simulink model "ng_pv_dynamic_dbus_p_4_ss_pmu"  (Simulink 8.8)
settings: Solver=ode4  StartTime=0.0  StopTime=inf  FixedStep=0.000125  RelTol=1e-3  EnableMultiTasking=on
PreLoadFcn:
  | Ts=125e-6;Core_Num = 0; np=1; nq=1; Vmin=.9;
PostLoadFcn:
  | Ts=125e-6;Core_Num = 0; np=1; nq=1; Vmin=.9;
InitFcn:
  | Ts=125e-6;Core_Num = 0; np=1; nq=1; Vmin=.9;
libraries: powerlib_meascontrol x180, rtio_generic_c37_118 x22, simulink x22, opal_lib x4, artemis x1, rtlab x1, powerlib x1
(part 4 of 4)

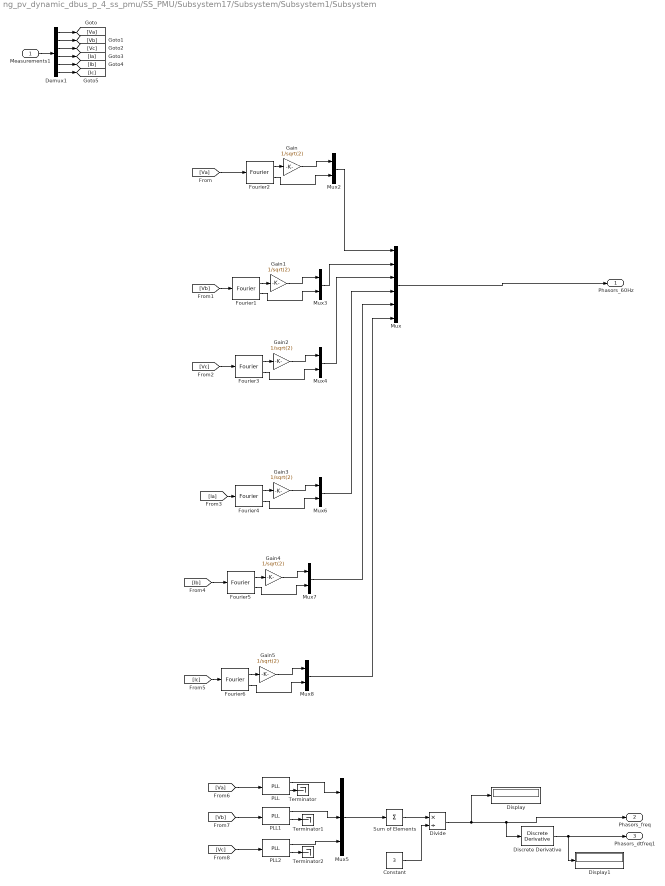
== system ng_pv_dynamic_dbus_p_4_ss_pmu/SS_PMU/Subsystem17/Subsystem/Subsystem1/Subsystem ==
  Measurements1 : Inport
  Constant : Constant  Value=3
  Demux1 : Demux  Outputs=6
  Discrete Derivative : simulink/Discrete/Discrete Derivative  gainval=1.0  ICPrevScaledInput=0.0  InputProcessing=Inherited  OutMin=[]  OutMax=[]  OutDataType=fixdt(1, 16)  OutScaling=2^-10  DoSatur=off
  Display : Display
  Display1 : Display
  Divide : Product  Inputs=*/
  Fourier{1..6} (6 alike) : powerlib_meascontrol/Measurements/Fourier  Freq=60  n=1  InInit=[0, 0]  Ts=Ts
  Gain{,1..5} (6 alike) : Gain  Gain=1/sqrt(2)
  Mux : Mux  Inputs=6
  Mux{2..4,6..8} (6 alike) : Mux  Inputs=2
  Mux5 : Mux  Inputs=3
  PLL : powerlib_meascontrol/PLL/PLL  Fmin=60  Par_Init=[0, 60]  ParK=[180, 3200, 1]  TcD=1.6e-4  MaxRateChangeFreq=12  FilterCutOffFreq=25  Ts=Ts  AGC=on
  PLL1 : powerlib_meascontrol/PLL/PLL  Fmin=60  Par_Init=[0, 60]  ParK=[180, 3200, 1]  TcD=1.6e-4  MaxRateChangeFreq=12  FilterCutOffFreq=25  Ts=Ts  AGC=on
  PLL2 : powerlib_meascontrol/PLL/PLL  Fmin=60  Par_Init=[0, 60]  ParK=[180, 3200, 1]  TcD=1.6e-4  MaxRateChangeFreq=12  FilterCutOffFreq=25  Ts=Ts  AGC=on
  Sum of Elements : Sum  Inputs=+
  Terminator : Terminator
  Terminator1 : Terminator
  Terminator2 : Terminator
  Phasors_60Hz : Outport
  Phasors_freq : Outport  Port=2
  Phasors_dtfreq1 : Outport  Port=3
  wires:
  Mux5/1 -> Sum of Elements/1
  PLL2/1 -> Mux5/3
  PLL1/1 -> Mux5/2
  PLL/1 -> Mux5/1
  PLL2/2 -> Terminator2/1
  PLL1/2 -> Terminator1/1
  PLL/2 -> Terminator/1
  [Vc] -> PLL2/1
  [Vb] -> PLL1/1
  [Va] -> PLL/1
  Discrete Derivative/1 -> Display1/1, Phasors_dtfreq1/1
  Mux3/1 -> Mux/2
  Mux2/1 -> Mux/1
  Demux1/2 -> [Vb]
  Measurements1/1 -> Demux1/1
  [Va] -> Fourier2/1
  Demux1/3 -> [Vc]
  Demux1/1 -> [Va]
  Mux7/1 -> Mux/5
  Mux4/1 -> Mux/3
  Mux/1 -> Phasors_60Hz/1
  Demux1/4 -> [Ia]
  Demux1/6 -> [Ic]
  Demux1/5 -> [Ib]
  Mux8/1 -> Mux/6
  Mux6/1 -> Mux/4
  Sum of Elements/1 -> Divide/1
  Divide/1 -> Display/1, Discrete Derivative/1, Phasors_freq/1
  Constant/1 -> Divide/2
  Fourier2/2 -> Mux2/2
  [Vc] -> Fourier3/1
  [Ia] -> Fourier4/1
  Fourier2/1 -> Gain/1
  Gain/1 -> Mux2/1
  [Vb] -> Fourier1/1
  Fourier1/2 -> Mux3/2
  Fourier1/1 -> Gain1/1
  Gain1/1 -> Mux3/1
  Fourier3/2 -> Mux4/2
  Fourier3/1 -> Gain2/1
  Gain2/1 -> Mux4/1
  Fourier4/2 -> Mux6/2
  Fourier4/1 -> Gain3/1
  Gain3/1 -> Mux6/1
  Fourier5/2 -> Mux7/2
  Fourier5/1 -> Gain4/1
  Gain4/1 -> Mux7/1
  Fourier6/2 -> Mux8/2
  Fourier6/1 -> Gain5/1
  Gain5/1 -> Mux8/1
  [Ic] -> Fourier6/1
  [Ib] -> Fourier5/1

== system ng_pv_dynamic_dbus_p_4_ss_pmu/SS_PMU/Subsystem18/Subsystem/Subsystem1/Degree to radian1 ==
  Degree : Inport
  Constant : Constant  Value=pi
  Constant1 : Constant  Value=180
  Divide : Product  Inputs=*/
  Product : Product  RndMeth=Zero
  Radian : Outport
  wires:
  Divide/1 -> Radian/1
  Degree/1 -> Product/1
  Constant1/1 -> Divide/2
  Product/1 -> Divide/1
  Constant/1 -> Product/2

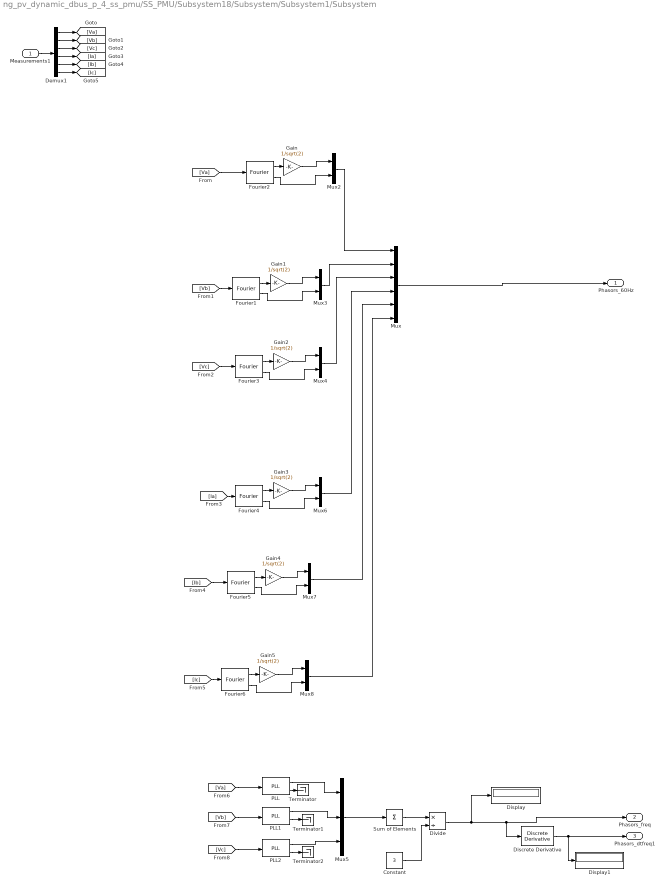
== system ng_pv_dynamic_dbus_p_4_ss_pmu/SS_PMU/Subsystem18/Subsystem/Subsystem1/Subsystem ==
  Measurements1 : Inport
  Constant : Constant  Value=3
  Demux1 : Demux  Outputs=6
  Discrete Derivative : simulink/Discrete/Discrete Derivative  gainval=1.0  ICPrevScaledInput=0.0  InputProcessing=Inherited  OutMin=[]  OutMax=[]  OutDataType=fixdt(1, 16)  OutScaling=2^-10  DoSatur=off
  Display : Display
  Display1 : Display
  Divide : Product  Inputs=*/
  Fourier{1..6} (6 alike) : powerlib_meascontrol/Measurements/Fourier  Freq=60  n=1  InInit=[0, 0]  Ts=Ts
  Gain{,1..5} (6 alike) : Gain  Gain=1/sqrt(2)
  Mux : Mux  Inputs=6
  Mux{2..4,6..8} (6 alike) : Mux  Inputs=2
  Mux5 : Mux  Inputs=3
  PLL : powerlib_meascontrol/PLL/PLL  Fmin=60  Par_Init=[0, 60]  ParK=[180, 3200, 1]  TcD=1.6e-4  MaxRateChangeFreq=12  FilterCutOffFreq=25  Ts=Ts  AGC=on
  PLL1 : powerlib_meascontrol/PLL/PLL  Fmin=60  Par_Init=[0, 60]  ParK=[180, 3200, 1]  TcD=1.6e-4  MaxRateChangeFreq=12  FilterCutOffFreq=25  Ts=Ts  AGC=on
  PLL2 : powerlib_meascontrol/PLL/PLL  Fmin=60  Par_Init=[0, 60]  ParK=[180, 3200, 1]  TcD=1.6e-4  MaxRateChangeFreq=12  FilterCutOffFreq=25  Ts=Ts  AGC=on
  Sum of Elements : Sum  Inputs=+
  Terminator : Terminator
  Terminator1 : Terminator
  Terminator2 : Terminator
  Phasors_60Hz : Outport
  Phasors_freq : Outport  Port=2
  Phasors_dtfreq1 : Outport  Port=3
  wires:
  Mux5/1 -> Sum of Elements/1
  PLL2/1 -> Mux5/3
  PLL1/1 -> Mux5/2
  PLL/1 -> Mux5/1
  PLL2/2 -> Terminator2/1
  PLL1/2 -> Terminator1/1
  PLL/2 -> Terminator/1
  [Vc] -> PLL2/1
  [Vb] -> PLL1/1
  [Va] -> PLL/1
  Discrete Derivative/1 -> Display1/1, Phasors_dtfreq1/1
  Mux3/1 -> Mux/2
  Mux2/1 -> Mux/1
  Demux1/2 -> [Vb]
  Measurements1/1 -> Demux1/1
  [Va] -> Fourier2/1
  Demux1/3 -> [Vc]
  Demux1/1 -> [Va]
  Mux7/1 -> Mux/5
  Mux4/1 -> Mux/3
  Mux/1 -> Phasors_60Hz/1
  Demux1/4 -> [Ia]
  Demux1/6 -> [Ic]
  Demux1/5 -> [Ib]
  Mux8/1 -> Mux/6
  Mux6/1 -> Mux/4
  Sum of Elements/1 -> Divide/1
  Divide/1 -> Display/1, Discrete Derivative/1, Phasors_freq/1
  Constant/1 -> Divide/2
  Fourier2/2 -> Mux2/2
  [Vc] -> Fourier3/1
  [Ia] -> Fourier4/1
  Fourier2/1 -> Gain/1
  Gain/1 -> Mux2/1
  [Vb] -> Fourier1/1
  Fourier1/2 -> Mux3/2
  Fourier1/1 -> Gain1/1
  Gain1/1 -> Mux3/1
  Fourier3/2 -> Mux4/2
  Fourier3/1 -> Gain2/1
  Gain2/1 -> Mux4/1
  Fourier4/2 -> Mux6/2
  Fourier4/1 -> Gain3/1
  Gain3/1 -> Mux6/1
  Fourier5/2 -> Mux7/2
  Fourier5/1 -> Gain4/1
  Gain4/1 -> Mux7/1
  Fourier6/2 -> Mux8/2
  Fourier6/1 -> Gain5/1
  Gain5/1 -> Mux8/1
  [Ic] -> Fourier6/1
  [Ib] -> Fourier5/1

== system ng_pv_dynamic_dbus_p_4_ss_pmu/SS_PMU/Subsystem19/Subsystem/Subsystem1/Degree to radian1 ==
  Degree : Inport
  Constant : Constant  Value=pi
  Constant1 : Constant  Value=180
  Divide : Product  Inputs=*/
  Product : Product  RndMeth=Zero
  Radian : Outport
  wires:
  Divide/1 -> Radian/1
  Degree/1 -> Product/1
  Constant1/1 -> Divide/2
  Product/1 -> Divide/1
  Constant/1 -> Product/2

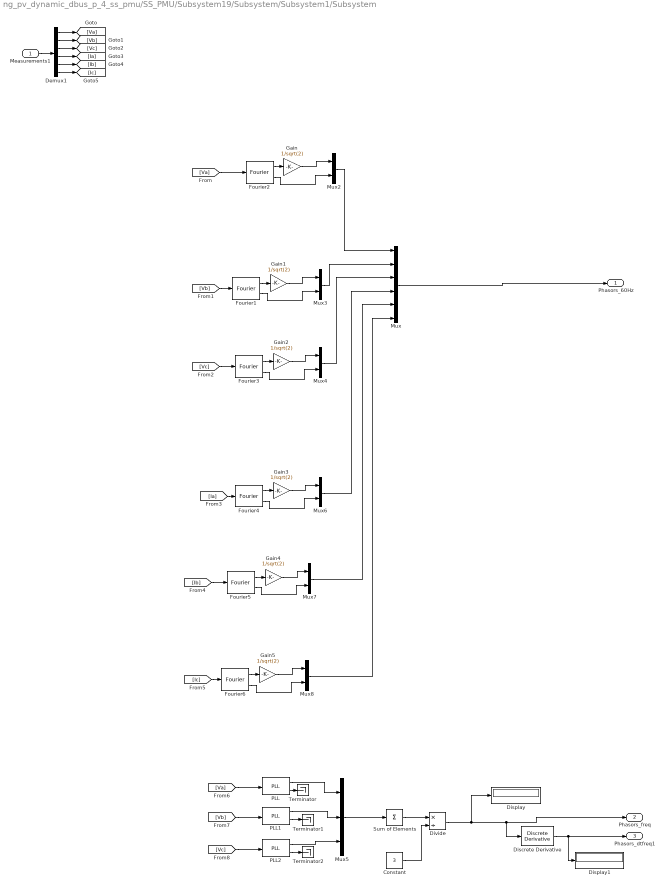
== system ng_pv_dynamic_dbus_p_4_ss_pmu/SS_PMU/Subsystem19/Subsystem/Subsystem1/Subsystem ==
  Measurements1 : Inport
  Constant : Constant  Value=3
  Demux1 : Demux  Outputs=6
  Discrete Derivative : simulink/Discrete/Discrete Derivative  gainval=1.0  ICPrevScaledInput=0.0  InputProcessing=Inherited  OutMin=[]  OutMax=[]  OutDataType=fixdt(1, 16)  OutScaling=2^-10  DoSatur=off
  Display : Display
  Display1 : Display
  Divide : Product  Inputs=*/
  Fourier{1..6} (6 alike) : powerlib_meascontrol/Measurements/Fourier  Freq=60  n=1  InInit=[0, 0]  Ts=Ts
  Gain{,1..5} (6 alike) : Gain  Gain=1/sqrt(2)
  Mux : Mux  Inputs=6
  Mux{2..4,6..8} (6 alike) : Mux  Inputs=2
  Mux5 : Mux  Inputs=3
  PLL : powerlib_meascontrol/PLL/PLL  Fmin=60  Par_Init=[0, 60]  ParK=[180, 3200, 1]  TcD=1.6e-4  MaxRateChangeFreq=12  FilterCutOffFreq=25  Ts=Ts  AGC=on
  PLL1 : powerlib_meascontrol/PLL/PLL  Fmin=60  Par_Init=[0, 60]  ParK=[180, 3200, 1]  TcD=1.6e-4  MaxRateChangeFreq=12  FilterCutOffFreq=25  Ts=Ts  AGC=on
  PLL2 : powerlib_meascontrol/PLL/PLL  Fmin=60  Par_Init=[0, 60]  ParK=[180, 3200, 1]  TcD=1.6e-4  MaxRateChangeFreq=12  FilterCutOffFreq=25  Ts=Ts  AGC=on
  Sum of Elements : Sum  Inputs=+
  Terminator : Terminator
  Terminator1 : Terminator
  Terminator2 : Terminator
  Phasors_60Hz : Outport
  Phasors_freq : Outport  Port=2
  Phasors_dtfreq1 : Outport  Port=3
  wires:
  Mux5/1 -> Sum of Elements/1
  PLL2/1 -> Mux5/3
  PLL1/1 -> Mux5/2
  PLL/1 -> Mux5/1
  PLL2/2 -> Terminator2/1
  PLL1/2 -> Terminator1/1
  PLL/2 -> Terminator/1
  [Vc] -> PLL2/1
  [Vb] -> PLL1/1
  [Va] -> PLL/1
  Discrete Derivative/1 -> Display1/1, Phasors_dtfreq1/1
  Mux3/1 -> Mux/2
  Mux2/1 -> Mux/1
  Demux1/2 -> [Vb]
  Measurements1/1 -> Demux1/1
  [Va] -> Fourier2/1
  Demux1/3 -> [Vc]
  Demux1/1 -> [Va]
  Mux7/1 -> Mux/5
  Mux4/1 -> Mux/3
  Mux/1 -> Phasors_60Hz/1
  Demux1/4 -> [Ia]
  Demux1/6 -> [Ic]
  Demux1/5 -> [Ib]
  Mux8/1 -> Mux/6
  Mux6/1 -> Mux/4
  Sum of Elements/1 -> Divide/1
  Divide/1 -> Display/1, Discrete Derivative/1, Phasors_freq/1
  Constant/1 -> Divide/2
  Fourier2/2 -> Mux2/2
  [Vc] -> Fourier3/1
  [Ia] -> Fourier4/1
  Fourier2/1 -> Gain/1
  Gain/1 -> Mux2/1
  [Vb] -> Fourier1/1
  Fourier1/2 -> Mux3/2
  Fourier1/1 -> Gain1/1
  Gain1/1 -> Mux3/1
  Fourier3/2 -> Mux4/2
  Fourier3/1 -> Gain2/1
  Gain2/1 -> Mux4/1
  Fourier4/2 -> Mux6/2
  Fourier4/1 -> Gain3/1
  Gain3/1 -> Mux6/1
  Fourier5/2 -> Mux7/2
  Fourier5/1 -> Gain4/1
  Gain4/1 -> Mux7/1
  Fourier6/2 -> Mux8/2
  Fourier6/1 -> Gain5/1
  Gain5/1 -> Mux8/1
  [Ic] -> Fourier6/1
  [Ib] -> Fourier5/1

== system ng_pv_dynamic_dbus_p_4_ss_pmu/SS_PMU/Subsystem2/Subsystem/Subsystem1/Degree to radian1 ==
  Degree : Inport
  Constant : Constant  Value=pi
  Constant1 : Constant  Value=180
  Divide : Product  Inputs=*/
  Product : Product  RndMeth=Zero
  Radian : Outport
  wires:
  Divide/1 -> Radian/1
  Degree/1 -> Product/1
  Constant1/1 -> Divide/2
  Product/1 -> Divide/1
  Constant/1 -> Product/2

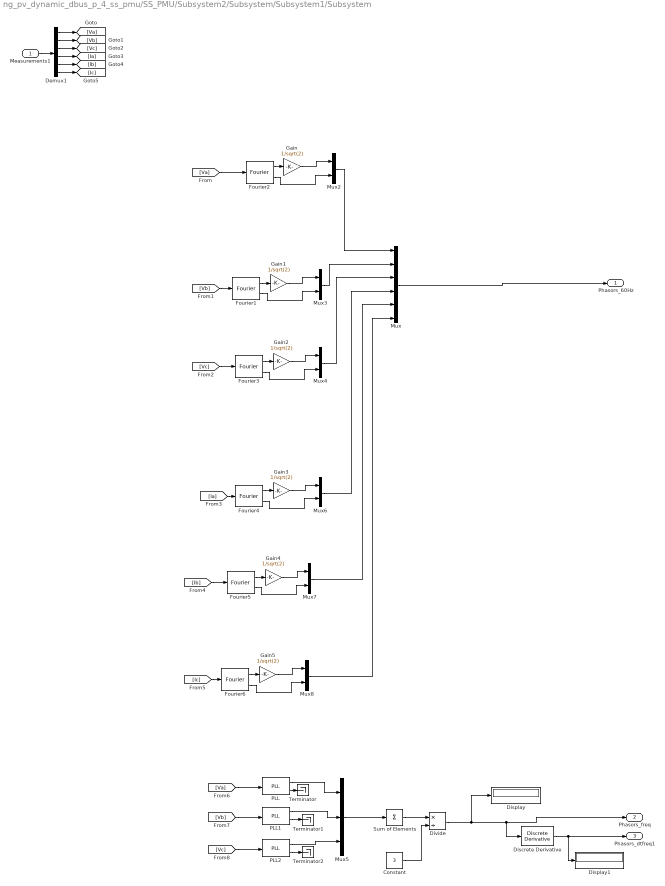
== system ng_pv_dynamic_dbus_p_4_ss_pmu/SS_PMU/Subsystem2/Subsystem/Subsystem1/Subsystem ==
  Measurements1 : Inport
  Constant : Constant  Value=3
  Demux1 : Demux  Outputs=6
  Discrete Derivative : simulink/Discrete/Discrete Derivative  gainval=1.0  ICPrevScaledInput=0.0  InputProcessing=Inherited  OutMin=[]  OutMax=[]  OutDataType=fixdt(1, 16)  OutScaling=2^-10  DoSatur=off
  Display : Display
  Display1 : Display
  Divide : Product  Inputs=*/
  Fourier{1..6} (6 alike) : powerlib_meascontrol/Measurements/Fourier  Freq=60  n=1  InInit=[0, 0]  Ts=Ts
  Gain{,1..5} (6 alike) : Gain  Gain=1/sqrt(2)
  Mux : Mux  Inputs=6
  Mux{2..4,6..8} (6 alike) : Mux  Inputs=2
  Mux5 : Mux  Inputs=3
  PLL : powerlib_meascontrol/PLL/PLL  Fmin=60  Par_Init=[0, 60]  ParK=[180, 3200, 1]  TcD=1.6e-4  MaxRateChangeFreq=12  FilterCutOffFreq=25  Ts=Ts  AGC=on
  PLL1 : powerlib_meascontrol/PLL/PLL  Fmin=60  Par_Init=[0, 60]  ParK=[180, 3200, 1]  TcD=1.6e-4  MaxRateChangeFreq=12  FilterCutOffFreq=25  Ts=Ts  AGC=on
  PLL2 : powerlib_meascontrol/PLL/PLL  Fmin=60  Par_Init=[0, 60]  ParK=[180, 3200, 1]  TcD=1.6e-4  MaxRateChangeFreq=12  FilterCutOffFreq=25  Ts=Ts  AGC=on
  Sum of Elements : Sum  Inputs=+
  Terminator : Terminator
  Terminator1 : Terminator
  Terminator2 : Terminator
  Phasors_60Hz : Outport
  Phasors_freq : Outport  Port=2
  Phasors_dtfreq1 : Outport  Port=3
  wires:
  Mux5/1 -> Sum of Elements/1
  PLL2/1 -> Mux5/3
  PLL1/1 -> Mux5/2
  PLL/1 -> Mux5/1
  PLL2/2 -> Terminator2/1
  PLL1/2 -> Terminator1/1
  PLL/2 -> Terminator/1
  [Vc] -> PLL2/1
  [Vb] -> PLL1/1
  [Va] -> PLL/1
  Discrete Derivative/1 -> Display1/1, Phasors_dtfreq1/1
  Mux3/1 -> Mux/2
  Mux2/1 -> Mux/1
  Demux1/2 -> [Vb]
  Measurements1/1 -> Demux1/1
  [Va] -> Fourier2/1
  Demux1/3 -> [Vc]
  Demux1/1 -> [Va]
  Mux7/1 -> Mux/5
  Mux4/1 -> Mux/3
  Mux/1 -> Phasors_60Hz/1
  Demux1/4 -> [Ia]
  Demux1/6 -> [Ic]
  Demux1/5 -> [Ib]
  Mux8/1 -> Mux/6
  Mux6/1 -> Mux/4
  Sum of Elements/1 -> Divide/1
  Divide/1 -> Display/1, Discrete Derivative/1, Phasors_freq/1
  Constant/1 -> Divide/2
  Fourier2/2 -> Mux2/2
  [Vc] -> Fourier3/1
  [Ia] -> Fourier4/1
  Fourier2/1 -> Gain/1
  Gain/1 -> Mux2/1
  [Vb] -> Fourier1/1
  Fourier1/2 -> Mux3/2
  Fourier1/1 -> Gain1/1
  Gain1/1 -> Mux3/1
  Fourier3/2 -> Mux4/2
  Fourier3/1 -> Gain2/1
  Gain2/1 -> Mux4/1
  Fourier4/2 -> Mux6/2
  Fourier4/1 -> Gain3/1
  Gain3/1 -> Mux6/1
  Fourier5/2 -> Mux7/2
  Fourier5/1 -> Gain4/1
  Gain4/1 -> Mux7/1
  Fourier6/2 -> Mux8/2
  Fourier6/1 -> Gain5/1
  Gain5/1 -> Mux8/1
  [Ic] -> Fourier6/1
  [Ib] -> Fourier5/1

== system ng_pv_dynamic_dbus_p_4_ss_pmu/SS_PMU/Subsystem20/Subsystem/Subsystem1/Degree to radian1 ==
  Degree : Inport
  Constant : Constant  Value=pi
  Constant1 : Constant  Value=180
  Divide : Product  Inputs=*/
  Product : Product  RndMeth=Zero
  Radian : Outport
  wires:
  Divide/1 -> Radian/1
  Degree/1 -> Product/1
  Constant1/1 -> Divide/2
  Product/1 -> Divide/1
  Constant/1 -> Product/2

== system ng_pv_dynamic_dbus_p_4_ss_pmu/SS_PMU/Subsystem20/Subsystem/Subsystem1/Subsystem ==
  Measurements1 : Inport
  Constant : Constant  Value=3
  Demux1 : Demux  Outputs=6
  Discrete Derivative : simulink/Discrete/Discrete Derivative  gainval=1.0  ICPrevScaledInput=0.0  InputProcessing=Inherited  OutMin=[]  OutMax=[]  OutDataType=fixdt(1, 16)  OutScaling=2^-10  DoSatur=off
  Display : Display
  Display1 : Display
  Divide : Product  Inputs=*/
  Fourier{1..6} (6 alike) : powerlib_meascontrol/Measurements/Fourier  Freq=60  n=1  InInit=[0, 0]  Ts=Ts
  Gain{,1..5} (6 alike) : Gain  Gain=1/sqrt(2)
  Mux : Mux  Inputs=6
  Mux{2..4,6..8} (6 alike) : Mux  Inputs=2
  Mux5 : Mux  Inputs=3
  PLL : powerlib_meascontrol/PLL/PLL  Fmin=60  Par_Init=[0, 60]  ParK=[180, 3200, 1]  TcD=1.6e-4  MaxRateChangeFreq=12  FilterCutOffFreq=25  Ts=Ts  AGC=on
  PLL1 : powerlib_meascontrol/PLL/PLL  Fmin=60  Par_Init=[0, 60]  ParK=[180, 3200, 1]  TcD=1.6e-4  MaxRateChangeFreq=12  FilterCutOffFreq=25  Ts=Ts  AGC=on
  PLL2 : powerlib_meascontrol/PLL/PLL  Fmin=60  Par_Init=[0, 60]  ParK=[180, 3200, 1]  TcD=1.6e-4  MaxRateChangeFreq=12  FilterCutOffFreq=25  Ts=Ts  AGC=on
  Sum of Elements : Sum  Inputs=+
  Terminator : Terminator
  Terminator1 : Terminator
  Terminator2 : Terminator
  Phasors_60Hz : Outport
  Phasors_freq : Outport  Port=2
  Phasors_dtfreq1 : Outport  Port=3
  wires:
  Mux5/1 -> Sum of Elements/1
  PLL2/1 -> Mux5/3
  PLL1/1 -> Mux5/2
  PLL/1 -> Mux5/1
  PLL2/2 -> Terminator2/1
  PLL1/2 -> Terminator1/1
  PLL/2 -> Terminator/1
  [Vc] -> PLL2/1
  [Vb] -> PLL1/1
  [Va] -> PLL/1
  Discrete Derivative/1 -> Display1/1, Phasors_dtfreq1/1
  Mux3/1 -> Mux/2
  Mux2/1 -> Mux/1
  Demux1/2 -> [Vb]
  Measurements1/1 -> Demux1/1
  [Va] -> Fourier2/1
  Demux1/3 -> [Vc]
  Demux1/1 -> [Va]
  Mux7/1 -> Mux/5
  Mux4/1 -> Mux/3
  Mux/1 -> Phasors_60Hz/1
  Demux1/4 -> [Ia]
  Demux1/6 -> [Ic]
  Demux1/5 -> [Ib]
  Mux8/1 -> Mux/6
  Mux6/1 -> Mux/4
  Sum of Elements/1 -> Divide/1
  Divide/1 -> Display/1, Discrete Derivative/1, Phasors_freq/1
  Constant/1 -> Divide/2
  Fourier2/2 -> Mux2/2
  [Vc] -> Fourier3/1
  [Ia] -> Fourier4/1
  Fourier2/1 -> Gain/1
  Gain/1 -> Mux2/1
  [Vb] -> Fourier1/1
  Fourier1/2 -> Mux3/2
  Fourier1/1 -> Gain1/1
  Gain1/1 -> Mux3/1
  Fourier3/2 -> Mux4/2
  Fourier3/1 -> Gain2/1
  Gain2/1 -> Mux4/1
  Fourier4/2 -> Mux6/2
  Fourier4/1 -> Gain3/1
  Gain3/1 -> Mux6/1
  Fourier5/2 -> Mux7/2
  Fourier5/1 -> Gain4/1
  Gain4/1 -> Mux7/1
  Fourier6/2 -> Mux8/2
  Fourier6/1 -> Gain5/1
  Gain5/1 -> Mux8/1
  [Ic] -> Fourier6/1
  [Ib] -> Fourier5/1

== system ng_pv_dynamic_dbus_p_4_ss_pmu/SS_PMU/Subsystem21/Subsystem/Subsystem1/Degree to radian1 ==
  Degree : Inport
  Constant : Constant  Value=pi
  Constant1 : Constant  Value=180
  Divide : Product  Inputs=*/
  Product : Product  RndMeth=Zero
  Radian : Outport
  wires:
  Divide/1 -> Radian/1
  Degree/1 -> Product/1
  Constant1/1 -> Divide/2
  Product/1 -> Divide/1
  Constant/1 -> Product/2

== system ng_pv_dynamic_dbus_p_4_ss_pmu/SS_PMU/Subsystem21/Subsystem/Subsystem1/Subsystem ==
  Measurements1 : Inport
  Constant : Constant  Value=3
  Demux1 : Demux  Outputs=6
  Discrete Derivative : simulink/Discrete/Discrete Derivative  gainval=1.0  ICPrevScaledInput=0.0  InputProcessing=Inherited  OutMin=[]  OutMax=[]  OutDataType=fixdt(1, 16)  OutScaling=2^-10  DoSatur=off
  Display : Display
  Display1 : Display
  Divide : Product  Inputs=*/
  Fourier{1..6} (6 alike) : powerlib_meascontrol/Measurements/Fourier  Freq=60  n=1  InInit=[0, 0]  Ts=Ts
  Gain{,1..5} (6 alike) : Gain  Gain=1/sqrt(2)
  Mux : Mux  Inputs=6
  Mux{2..4,6..8} (6 alike) : Mux  Inputs=2
  Mux5 : Mux  Inputs=3
  PLL : powerlib_meascontrol/PLL/PLL  Fmin=60  Par_Init=[0, 60]  ParK=[180, 3200, 1]  TcD=1.6e-4  MaxRateChangeFreq=12  FilterCutOffFreq=25  Ts=Ts  AGC=on
  PLL1 : powerlib_meascontrol/PLL/PLL  Fmin=60  Par_Init=[0, 60]  ParK=[180, 3200, 1]  TcD=1.6e-4  MaxRateChangeFreq=12  FilterCutOffFreq=25  Ts=Ts  AGC=on
  PLL2 : powerlib_meascontrol/PLL/PLL  Fmin=60  Par_Init=[0, 60]  ParK=[180, 3200, 1]  TcD=1.6e-4  MaxRateChangeFreq=12  FilterCutOffFreq=25  Ts=Ts  AGC=on
  Sum of Elements : Sum  Inputs=+
  Terminator : Terminator
  Terminator1 : Terminator
  Terminator2 : Terminator
  Phasors_60Hz : Outport
  Phasors_freq : Outport  Port=2
  Phasors_dtfreq1 : Outport  Port=3
  wires:
  Mux5/1 -> Sum of Elements/1
  PLL2/1 -> Mux5/3
  PLL1/1 -> Mux5/2
  PLL/1 -> Mux5/1
  PLL2/2 -> Terminator2/1
  PLL1/2 -> Terminator1/1
  PLL/2 -> Terminator/1
  [Vc] -> PLL2/1
  [Vb] -> PLL1/1
  [Va] -> PLL/1
  Discrete Derivative/1 -> Display1/1, Phasors_dtfreq1/1
  Mux3/1 -> Mux/2
  Mux2/1 -> Mux/1
  Demux1/2 -> [Vb]
  Measurements1/1 -> Demux1/1
  [Va] -> Fourier2/1
  Demux1/3 -> [Vc]
  Demux1/1 -> [Va]
  Mux7/1 -> Mux/5
  Mux4/1 -> Mux/3
  Mux/1 -> Phasors_60Hz/1
  Demux1/4 -> [Ia]
  Demux1/6 -> [Ic]
  Demux1/5 -> [Ib]
  Mux8/1 -> Mux/6
  Mux6/1 -> Mux/4
  Sum of Elements/1 -> Divide/1
  Divide/1 -> Display/1, Discrete Derivative/1, Phasors_freq/1
  Constant/1 -> Divide/2
  Fourier2/2 -> Mux2/2
  [Vc] -> Fourier3/1
  [Ia] -> Fourier4/1
  Fourier2/1 -> Gain/1
  Gain/1 -> Mux2/1
  [Vb] -> Fourier1/1
  Fourier1/2 -> Mux3/2
  Fourier1/1 -> Gain1/1
  Gain1/1 -> Mux3/1
  Fourier3/2 -> Mux4/2
  Fourier3/1 -> Gain2/1
  Gain2/1 -> Mux4/1
  Fourier4/2 -> Mux6/2
  Fourier4/1 -> Gain3/1
  Gain3/1 -> Mux6/1
  Fourier5/2 -> Mux7/2
  Fourier5/1 -> Gain4/1
  Gain4/1 -> Mux7/1
  Fourier6/2 -> Mux8/2
  Fourier6/1 -> Gain5/1
  Gain5/1 -> Mux8/1
  [Ic] -> Fourier6/1
  [Ib] -> Fourier5/1

== system ng_pv_dynamic_dbus_p_4_ss_pmu/SS_PMU/Subsystem22/Subsystem/Subsystem1/Degree to radian1 ==
  Degree : Inport
  Constant : Constant  Value=pi
  Constant1 : Constant  Value=180
  Divide : Product  Inputs=*/
  Product : Product  RndMeth=Zero
  Radian : Outport
  wires:
  Divide/1 -> Radian/1
  Degree/1 -> Product/1
  Constant1/1 -> Divide/2
  Product/1 -> Divide/1
  Constant/1 -> Product/2

== system ng_pv_dynamic_dbus_p_4_ss_pmu/SS_PMU/Subsystem22/Subsystem/Subsystem1/Subsystem ==
  Measurements1 : Inport
  Constant : Constant  Value=3
  Demux1 : Demux  Outputs=6
  Discrete Derivative : simulink/Discrete/Discrete Derivative  gainval=1.0  ICPrevScaledInput=0.0  InputProcessing=Inherited  OutMin=[]  OutMax=[]  OutDataType=fixdt(1, 16)  OutScaling=2^-10  DoSatur=off
  Display : Display
  Display1 : Display
  Divide : Product  Inputs=*/
  Fourier{1..6} (6 alike) : powerlib_meascontrol/Measurements/Fourier  Freq=60  n=1  InInit=[0, 0]  Ts=Ts
  Gain{,1..5} (6 alike) : Gain  Gain=1/sqrt(2)
  Mux : Mux  Inputs=6
  Mux{2..4,6..8} (6 alike) : Mux  Inputs=2
  Mux5 : Mux  Inputs=3
  PLL : powerlib_meascontrol/PLL/PLL  Fmin=60  Par_Init=[0, 60]  ParK=[180, 3200, 1]  TcD=1.6e-4  MaxRateChangeFreq=12  FilterCutOffFreq=25  Ts=Ts  AGC=on
  PLL1 : powerlib_meascontrol/PLL/PLL  Fmin=60  Par_Init=[0, 60]  ParK=[180, 3200, 1]  TcD=1.6e-4  MaxRateChangeFreq=12  FilterCutOffFreq=25  Ts=Ts  AGC=on
  PLL2 : powerlib_meascontrol/PLL/PLL  Fmin=60  Par_Init=[0, 60]  ParK=[180, 3200, 1]  TcD=1.6e-4  MaxRateChangeFreq=12  FilterCutOffFreq=25  Ts=Ts  AGC=on
  Sum of Elements : Sum  Inputs=+
  Terminator : Terminator
  Terminator1 : Terminator
  Terminator2 : Terminator
  Phasors_60Hz : Outport
  Phasors_freq : Outport  Port=2
  Phasors_dtfreq1 : Outport  Port=3
  wires:
  Mux5/1 -> Sum of Elements/1
  PLL2/1 -> Mux5/3
  PLL1/1 -> Mux5/2
  PLL/1 -> Mux5/1
  PLL2/2 -> Terminator2/1
  PLL1/2 -> Terminator1/1
  PLL/2 -> Terminator/1
  [Vc] -> PLL2/1
  [Vb] -> PLL1/1
  [Va] -> PLL/1
  Discrete Derivative/1 -> Display1/1, Phasors_dtfreq1/1
  Mux3/1 -> Mux/2
  Mux2/1 -> Mux/1
  Demux1/2 -> [Vb]
  Measurements1/1 -> Demux1/1
  [Va] -> Fourier2/1
  Demux1/3 -> [Vc]
  Demux1/1 -> [Va]
  Mux7/1 -> Mux/5
  Mux4/1 -> Mux/3
  Mux/1 -> Phasors_60Hz/1
  Demux1/4 -> [Ia]
  Demux1/6 -> [Ic]
  Demux1/5 -> [Ib]
  Mux8/1 -> Mux/6
  Mux6/1 -> Mux/4
  Sum of Elements/1 -> Divide/1
  Divide/1 -> Display/1, Discrete Derivative/1, Phasors_freq/1
  Constant/1 -> Divide/2
  Fourier2/2 -> Mux2/2
  [Vc] -> Fourier3/1
  [Ia] -> Fourier4/1
  Fourier2/1 -> Gain/1
  Gain/1 -> Mux2/1
  [Vb] -> Fourier1/1
  Fourier1/2 -> Mux3/2
  Fourier1/1 -> Gain1/1
  Gain1/1 -> Mux3/1
  Fourier3/2 -> Mux4/2
  Fourier3/1 -> Gain2/1
  Gain2/1 -> Mux4/1
  Fourier4/2 -> Mux6/2
  Fourier4/1 -> Gain3/1
  Gain3/1 -> Mux6/1
  Fourier5/2 -> Mux7/2
  Fourier5/1 -> Gain4/1
  Gain4/1 -> Mux7/1
  Fourier6/2 -> Mux8/2
  Fourier6/1 -> Gain5/1
  Gain5/1 -> Mux8/1
  [Ic] -> Fourier6/1
  [Ib] -> Fourier5/1

== system ng_pv_dynamic_dbus_p_4_ss_pmu/SS_PMU/Subsystem3/Subsystem/Subsystem1/Degree to radian1 ==
  Degree : Inport
  Constant : Constant  Value=pi
  Constant1 : Constant  Value=180
  Divide : Product  Inputs=*/
  Product : Product  RndMeth=Zero
  Radian : Outport
  wires:
  Divide/1 -> Radian/1
  Degree/1 -> Product/1
  Constant1/1 -> Divide/2
  Product/1 -> Divide/1
  Constant/1 -> Product/2

== system ng_pv_dynamic_dbus_p_4_ss_pmu/SS_PMU/Subsystem3/Subsystem/Subsystem1/Subsystem ==
  Measurements1 : Inport
  Constant : Constant  Value=3
  Demux1 : Demux  Outputs=6
  Discrete Derivative : simulink/Discrete/Discrete Derivative  gainval=1.0  ICPrevScaledInput=0.0  InputProcessing=Inherited  OutMin=[]  OutMax=[]  OutDataType=fixdt(1, 16)  OutScaling=2^-10  DoSatur=off
  Display : Display
  Display1 : Display
  Divide : Product  Inputs=*/
  Fourier{1..6} (6 alike) : powerlib_meascontrol/Measurements/Fourier  Freq=60  n=1  InInit=[0, 0]  Ts=Ts
  Gain{,1..5} (6 alike) : Gain  Gain=1/sqrt(2)
  Mux : Mux  Inputs=6
  Mux{2..4,6..8} (6 alike) : Mux  Inputs=2
  Mux5 : Mux  Inputs=3
  PLL : powerlib_meascontrol/PLL/PLL  Fmin=60  Par_Init=[0, 60]  ParK=[180, 3200, 1]  TcD=1.6e-4  MaxRateChangeFreq=12  FilterCutOffFreq=25  Ts=Ts  AGC=on
  PLL1 : powerlib_meascontrol/PLL/PLL  Fmin=60  Par_Init=[0, 60]  ParK=[180, 3200, 1]  TcD=1.6e-4  MaxRateChangeFreq=12  FilterCutOffFreq=25  Ts=Ts  AGC=on
  PLL2 : powerlib_meascontrol/PLL/PLL  Fmin=60  Par_Init=[0, 60]  ParK=[180, 3200, 1]  TcD=1.6e-4  MaxRateChangeFreq=12  FilterCutOffFreq=25  Ts=Ts  AGC=on
  Sum of Elements : Sum  Inputs=+
  Terminator : Terminator
  Terminator1 : Terminator
  Terminator2 : Terminator
  Phasors_60Hz : Outport
  Phasors_freq : Outport  Port=2
  Phasors_dtfreq1 : Outport  Port=3
  wires:
  Mux5/1 -> Sum of Elements/1
  PLL2/1 -> Mux5/3
  PLL1/1 -> Mux5/2
  PLL/1 -> Mux5/1
  PLL2/2 -> Terminator2/1
  PLL1/2 -> Terminator1/1
  PLL/2 -> Terminator/1
  [Vc] -> PLL2/1
  [Vb] -> PLL1/1
  [Va] -> PLL/1
  Discrete Derivative/1 -> Display1/1, Phasors_dtfreq1/1
  Mux3/1 -> Mux/2
  Mux2/1 -> Mux/1
  Demux1/2 -> [Vb]
  Measurements1/1 -> Demux1/1
  [Va] -> Fourier2/1
  Demux1/3 -> [Vc]
  Demux1/1 -> [Va]
  Mux7/1 -> Mux/5
  Mux4/1 -> Mux/3
  Mux/1 -> Phasors_60Hz/1
  Demux1/4 -> [Ia]
  Demux1/6 -> [Ic]
  Demux1/5 -> [Ib]
  Mux8/1 -> Mux/6
  Mux6/1 -> Mux/4
  Sum of Elements/1 -> Divide/1
  Divide/1 -> Display/1, Discrete Derivative/1, Phasors_freq/1
  Constant/1 -> Divide/2
  Fourier2/2 -> Mux2/2
  [Vc] -> Fourier3/1
  [Ia] -> Fourier4/1
  Fourier2/1 -> Gain/1
  Gain/1 -> Mux2/1
  [Vb] -> Fourier1/1
  Fourier1/2 -> Mux3/2
  Fourier1/1 -> Gain1/1
  Gain1/1 -> Mux3/1
  Fourier3/2 -> Mux4/2
  Fourier3/1 -> Gain2/1
  Gain2/1 -> Mux4/1
  Fourier4/2 -> Mux6/2
  Fourier4/1 -> Gain3/1
  Gain3/1 -> Mux6/1
  Fourier5/2 -> Mux7/2
  Fourier5/1 -> Gain4/1
  Gain4/1 -> Mux7/1
  Fourier6/2 -> Mux8/2
  Fourier6/1 -> Gain5/1
  Gain5/1 -> Mux8/1
  [Ic] -> Fourier6/1
  [Ib] -> Fourier5/1

== system ng_pv_dynamic_dbus_p_4_ss_pmu/SS_PMU/Subsystem4/Subsystem/Subsystem1/Degree to radian1 ==
  Degree : Inport
  Constant : Constant  Value=pi
  Constant1 : Constant  Value=180
  Divide : Product  Inputs=*/
  Product : Product  RndMeth=Zero
  Radian : Outport
  wires:
  Divide/1 -> Radian/1
  Degree/1 -> Product/1
  Constant1/1 -> Divide/2
  Product/1 -> Divide/1
  Constant/1 -> Product/2

== system ng_pv_dynamic_dbus_p_4_ss_pmu/SS_PMU/Subsystem4/Subsystem/Subsystem1/Subsystem ==
  Measurements1 : Inport
  Constant : Constant  Value=3
  Demux1 : Demux  Outputs=6
  Discrete Derivative : simulink/Discrete/Discrete Derivative  gainval=1.0  ICPrevScaledInput=0.0  InputProcessing=Inherited  OutMin=[]  OutMax=[]  OutDataType=fixdt(1, 16)  OutScaling=2^-10  DoSatur=off
  Display : Display
  Display1 : Display
  Divide : Product  Inputs=*/
  Fourier{1..6} (6 alike) : powerlib_meascontrol/Measurements/Fourier  Freq=60  n=1  InInit=[0, 0]  Ts=Ts
  Gain{,1..5} (6 alike) : Gain  Gain=1/sqrt(2)
  Mux : Mux  Inputs=6
  Mux{2..4,6..8} (6 alike) : Mux  Inputs=2
  Mux5 : Mux  Inputs=3
  PLL : powerlib_meascontrol/PLL/PLL  Fmin=60  Par_Init=[0, 60]  ParK=[180, 3200, 1]  TcD=1.6e-4  MaxRateChangeFreq=12  FilterCutOffFreq=25  Ts=Ts  AGC=on
  PLL1 : powerlib_meascontrol/PLL/PLL  Fmin=60  Par_Init=[0, 60]  ParK=[180, 3200, 1]  TcD=1.6e-4  MaxRateChangeFreq=12  FilterCutOffFreq=25  Ts=Ts  AGC=on
  PLL2 : powerlib_meascontrol/PLL/PLL  Fmin=60  Par_Init=[0, 60]  ParK=[180, 3200, 1]  TcD=1.6e-4  MaxRateChangeFreq=12  FilterCutOffFreq=25  Ts=Ts  AGC=on
  Sum of Elements : Sum  Inputs=+
  Terminator : Terminator
  Terminator1 : Terminator
  Terminator2 : Terminator
  Phasors_60Hz : Outport
  Phasors_freq : Outport  Port=2
  Phasors_dtfreq1 : Outport  Port=3
  wires:
  Mux5/1 -> Sum of Elements/1
  PLL2/1 -> Mux5/3
  PLL1/1 -> Mux5/2
  PLL/1 -> Mux5/1
  PLL2/2 -> Terminator2/1
  PLL1/2 -> Terminator1/1
  PLL/2 -> Terminator/1
  [Vc] -> PLL2/1
  [Vb] -> PLL1/1
  [Va] -> PLL/1
  Discrete Derivative/1 -> Display1/1, Phasors_dtfreq1/1
  Mux3/1 -> Mux/2
  Mux2/1 -> Mux/1
  Demux1/2 -> [Vb]
  Measurements1/1 -> Demux1/1
  [Va] -> Fourier2/1
  Demux1/3 -> [Vc]
  Demux1/1 -> [Va]
  Mux7/1 -> Mux/5
  Mux4/1 -> Mux/3
  Mux/1 -> Phasors_60Hz/1
  Demux1/4 -> [Ia]
  Demux1/6 -> [Ic]
  Demux1/5 -> [Ib]
  Mux8/1 -> Mux/6
  Mux6/1 -> Mux/4
  Sum of Elements/1 -> Divide/1
  Divide/1 -> Display/1, Discrete Derivative/1, Phasors_freq/1
  Constant/1 -> Divide/2
  Fourier2/2 -> Mux2/2
  [Vc] -> Fourier3/1
  [Ia] -> Fourier4/1
  Fourier2/1 -> Gain/1
  Gain/1 -> Mux2/1
  [Vb] -> Fourier1/1
  Fourier1/2 -> Mux3/2
  Fourier1/1 -> Gain1/1
  Gain1/1 -> Mux3/1
  Fourier3/2 -> Mux4/2
  Fourier3/1 -> Gain2/1
  Gain2/1 -> Mux4/1
  Fourier4/2 -> Mux6/2
  Fourier4/1 -> Gain3/1
  Gain3/1 -> Mux6/1
  Fourier5/2 -> Mux7/2
  Fourier5/1 -> Gain4/1
  Gain4/1 -> Mux7/1
  Fourier6/2 -> Mux8/2
  Fourier6/1 -> Gain5/1
  Gain5/1 -> Mux8/1
  [Ic] -> Fourier6/1
  [Ib] -> Fourier5/1

== system ng_pv_dynamic_dbus_p_4_ss_pmu/SS_PMU/Subsystem5/Subsystem/Subsystem1/Degree to radian1 ==
  Degree : Inport
  Constant : Constant  Value=pi
  Constant1 : Constant  Value=180
  Divide : Product  Inputs=*/
  Product : Product  RndMeth=Zero
  Radian : Outport
  wires:
  Divide/1 -> Radian/1
  Degree/1 -> Product/1
  Constant1/1 -> Divide/2
  Product/1 -> Divide/1
  Constant/1 -> Product/2

== system ng_pv_dynamic_dbus_p_4_ss_pmu/SS_PMU/Subsystem5/Subsystem/Subsystem1/Subsystem ==
  Measurements1 : Inport
  Constant : Constant  Value=3
  Demux1 : Demux  Outputs=6
  Discrete Derivative : simulink/Discrete/Discrete Derivative  gainval=1.0  ICPrevScaledInput=0.0  InputProcessing=Inherited  OutMin=[]  OutMax=[]  OutDataType=fixdt(1, 16)  OutScaling=2^-10  DoSatur=off
  Display : Display
  Display1 : Display
  Divide : Product  Inputs=*/
  Fourier{1..6} (6 alike) : powerlib_meascontrol/Measurements/Fourier  Freq=60  n=1  InInit=[0, 0]  Ts=Ts
  Gain{,1..5} (6 alike) : Gain  Gain=1/sqrt(2)
  Mux : Mux  Inputs=6
  Mux{2..4,6..8} (6 alike) : Mux  Inputs=2
  Mux5 : Mux  Inputs=3
  PLL : powerlib_meascontrol/PLL/PLL  Fmin=60  Par_Init=[0, 60]  ParK=[180, 3200, 1]  TcD=1.6e-4  MaxRateChangeFreq=12  FilterCutOffFreq=25  Ts=Ts  AGC=on
  PLL1 : powerlib_meascontrol/PLL/PLL  Fmin=60  Par_Init=[0, 60]  ParK=[180, 3200, 1]  TcD=1.6e-4  MaxRateChangeFreq=12  FilterCutOffFreq=25  Ts=Ts  AGC=on
  PLL2 : powerlib_meascontrol/PLL/PLL  Fmin=60  Par_Init=[0, 60]  ParK=[180, 3200, 1]  TcD=1.6e-4  MaxRateChangeFreq=12  FilterCutOffFreq=25  Ts=Ts  AGC=on
  Sum of Elements : Sum  Inputs=+
  Terminator : Terminator
  Terminator1 : Terminator
  Terminator2 : Terminator
  Phasors_60Hz : Outport
  Phasors_freq : Outport  Port=2
  Phasors_dtfreq1 : Outport  Port=3
  wires:
  Mux5/1 -> Sum of Elements/1
  PLL2/1 -> Mux5/3
  PLL1/1 -> Mux5/2
  PLL/1 -> Mux5/1
  PLL2/2 -> Terminator2/1
  PLL1/2 -> Terminator1/1
  PLL/2 -> Terminator/1
  [Vc] -> PLL2/1
  [Vb] -> PLL1/1
  [Va] -> PLL/1
  Discrete Derivative/1 -> Display1/1, Phasors_dtfreq1/1
  Mux3/1 -> Mux/2
  Mux2/1 -> Mux/1
  Demux1/2 -> [Vb]
  Measurements1/1 -> Demux1/1
  [Va] -> Fourier2/1
  Demux1/3 -> [Vc]
  Demux1/1 -> [Va]
  Mux7/1 -> Mux/5
  Mux4/1 -> Mux/3
  Mux/1 -> Phasors_60Hz/1
  Demux1/4 -> [Ia]
  Demux1/6 -> [Ic]
  Demux1/5 -> [Ib]
  Mux8/1 -> Mux/6
  Mux6/1 -> Mux/4
  Sum of Elements/1 -> Divide/1
  Divide/1 -> Display/1, Discrete Derivative/1, Phasors_freq/1
  Constant/1 -> Divide/2
  Fourier2/2 -> Mux2/2
  [Vc] -> Fourier3/1
  [Ia] -> Fourier4/1
  Fourier2/1 -> Gain/1
  Gain/1 -> Mux2/1
  [Vb] -> Fourier1/1
  Fourier1/2 -> Mux3/2
  Fourier1/1 -> Gain1/1
  Gain1/1 -> Mux3/1
  Fourier3/2 -> Mux4/2
  Fourier3/1 -> Gain2/1
  Gain2/1 -> Mux4/1
  Fourier4/2 -> Mux6/2
  Fourier4/1 -> Gain3/1
  Gain3/1 -> Mux6/1
  Fourier5/2 -> Mux7/2
  Fourier5/1 -> Gain4/1
  Gain4/1 -> Mux7/1
  Fourier6/2 -> Mux8/2
  Fourier6/1 -> Gain5/1
  Gain5/1 -> Mux8/1
  [Ic] -> Fourier6/1
  [Ib] -> Fourier5/1

== system ng_pv_dynamic_dbus_p_4_ss_pmu/SS_PMU/Subsystem6/Subsystem/Subsystem1/Degree to radian1 ==
  Degree : Inport
  Constant : Constant  Value=pi
  Constant1 : Constant  Value=180
  Divide : Product  Inputs=*/
  Product : Product  RndMeth=Zero
  Radian : Outport
  wires:
  Divide/1 -> Radian/1
  Degree/1 -> Product/1
  Constant1/1 -> Divide/2
  Product/1 -> Divide/1
  Constant/1 -> Product/2

== system ng_pv_dynamic_dbus_p_4_ss_pmu/SS_PMU/Subsystem6/Subsystem/Subsystem1/Subsystem ==
  Measurements1 : Inport
  Constant : Constant  Value=3
  Demux1 : Demux  Outputs=6
  Discrete Derivative : simulink/Discrete/Discrete Derivative  gainval=1.0  ICPrevScaledInput=0.0  InputProcessing=Inherited  OutMin=[]  OutMax=[]  OutDataType=fixdt(1, 16)  OutScaling=2^-10  DoSatur=off
  Display : Display
  Display1 : Display
  Divide : Product  Inputs=*/
  Fourier{1..6} (6 alike) : powerlib_meascontrol/Measurements/Fourier  Freq=60  n=1  InInit=[0, 0]  Ts=Ts
  Gain{,1..5} (6 alike) : Gain  Gain=1/sqrt(2)
  Mux : Mux  Inputs=6
  Mux{2..4,6..8} (6 alike) : Mux  Inputs=2
  Mux5 : Mux  Inputs=3
  PLL : powerlib_meascontrol/PLL/PLL  Fmin=60  Par_Init=[0, 60]  ParK=[180, 3200, 1]  TcD=1.6e-4  MaxRateChangeFreq=12  FilterCutOffFreq=25  Ts=Ts  AGC=on
  PLL1 : powerlib_meascontrol/PLL/PLL  Fmin=60  Par_Init=[0, 60]  ParK=[180, 3200, 1]  TcD=1.6e-4  MaxRateChangeFreq=12  FilterCutOffFreq=25  Ts=Ts  AGC=on
  PLL2 : powerlib_meascontrol/PLL/PLL  Fmin=60  Par_Init=[0, 60]  ParK=[180, 3200, 1]  TcD=1.6e-4  MaxRateChangeFreq=12  FilterCutOffFreq=25  Ts=Ts  AGC=on
  Sum of Elements : Sum  Inputs=+
  Terminator : Terminator
  Terminator1 : Terminator
  Terminator2 : Terminator
  Phasors_60Hz : Outport
  Phasors_freq : Outport  Port=2
  Phasors_dtfreq1 : Outport  Port=3
  wires:
  Mux5/1 -> Sum of Elements/1
  PLL2/1 -> Mux5/3
  PLL1/1 -> Mux5/2
  PLL/1 -> Mux5/1
  PLL2/2 -> Terminator2/1
  PLL1/2 -> Terminator1/1
  PLL/2 -> Terminator/1
  [Vc] -> PLL2/1
  [Vb] -> PLL1/1
  [Va] -> PLL/1
  Discrete Derivative/1 -> Display1/1, Phasors_dtfreq1/1
  Mux3/1 -> Mux/2
  Mux2/1 -> Mux/1
  Demux1/2 -> [Vb]
  Measurements1/1 -> Demux1/1
  [Va] -> Fourier2/1
  Demux1/3 -> [Vc]
  Demux1/1 -> [Va]
  Mux7/1 -> Mux/5
  Mux4/1 -> Mux/3
  Mux/1 -> Phasors_60Hz/1
  Demux1/4 -> [Ia]
  Demux1/6 -> [Ic]
  Demux1/5 -> [Ib]
  Mux8/1 -> Mux/6
  Mux6/1 -> Mux/4
  Sum of Elements/1 -> Divide/1
  Divide/1 -> Display/1, Discrete Derivative/1, Phasors_freq/1
  Constant/1 -> Divide/2
  Fourier2/2 -> Mux2/2
  [Vc] -> Fourier3/1
  [Ia] -> Fourier4/1
  Fourier2/1 -> Gain/1
  Gain/1 -> Mux2/1
  [Vb] -> Fourier1/1
  Fourier1/2 -> Mux3/2
  Fourier1/1 -> Gain1/1
  Gain1/1 -> Mux3/1
  Fourier3/2 -> Mux4/2
  Fourier3/1 -> Gain2/1
  Gain2/1 -> Mux4/1
  Fourier4/2 -> Mux6/2
  Fourier4/1 -> Gain3/1
  Gain3/1 -> Mux6/1
  Fourier5/2 -> Mux7/2
  Fourier5/1 -> Gain4/1
  Gain4/1 -> Mux7/1
  Fourier6/2 -> Mux8/2
  Fourier6/1 -> Gain5/1
  Gain5/1 -> Mux8/1
  [Ic] -> Fourier6/1
  [Ib] -> Fourier5/1

== system ng_pv_dynamic_dbus_p_4_ss_pmu/SS_PMU/Subsystem7/Subsystem/Subsystem1/Degree to radian1 ==
  Degree : Inport
  Constant : Constant  Value=pi
  Constant1 : Constant  Value=180
  Divide : Product  Inputs=*/
  Product : Product  RndMeth=Zero
  Radian : Outport
  wires:
  Divide/1 -> Radian/1
  Degree/1 -> Product/1
  Constant1/1 -> Divide/2
  Product/1 -> Divide/1
  Constant/1 -> Product/2

== system ng_pv_dynamic_dbus_p_4_ss_pmu/SS_PMU/Subsystem7/Subsystem/Subsystem1/Subsystem ==
  Measurements1 : Inport
  Constant : Constant  Value=3
  Demux1 : Demux  Outputs=6
  Discrete Derivative : simulink/Discrete/Discrete Derivative  gainval=1.0  ICPrevScaledInput=0.0  InputProcessing=Inherited  OutMin=[]  OutMax=[]  OutDataType=fixdt(1, 16)  OutScaling=2^-10  DoSatur=off
  Display : Display
  Display1 : Display
  Divide : Product  Inputs=*/
  Fourier{1..6} (6 alike) : powerlib_meascontrol/Measurements/Fourier  Freq=60  n=1  InInit=[0, 0]  Ts=Ts
  Gain{,1..5} (6 alike) : Gain  Gain=1/sqrt(2)
  Mux : Mux  Inputs=6
  Mux{2..4,6..8} (6 alike) : Mux  Inputs=2
  Mux5 : Mux  Inputs=3
  PLL : powerlib_meascontrol/PLL/PLL  Fmin=60  Par_Init=[0, 60]  ParK=[180, 3200, 1]  TcD=1.6e-4  MaxRateChangeFreq=12  FilterCutOffFreq=25  Ts=Ts  AGC=on
  PLL1 : powerlib_meascontrol/PLL/PLL  Fmin=60  Par_Init=[0, 60]  ParK=[180, 3200, 1]  TcD=1.6e-4  MaxRateChangeFreq=12  FilterCutOffFreq=25  Ts=Ts  AGC=on
  PLL2 : powerlib_meascontrol/PLL/PLL  Fmin=60  Par_Init=[0, 60]  ParK=[180, 3200, 1]  TcD=1.6e-4  MaxRateChangeFreq=12  FilterCutOffFreq=25  Ts=Ts  AGC=on
  Sum of Elements : Sum  Inputs=+
  Terminator : Terminator
  Terminator1 : Terminator
  Terminator2 : Terminator
  Phasors_60Hz : Outport
  Phasors_freq : Outport  Port=2
  Phasors_dtfreq1 : Outport  Port=3
  wires:
  Mux5/1 -> Sum of Elements/1
  PLL2/1 -> Mux5/3
  PLL1/1 -> Mux5/2
  PLL/1 -> Mux5/1
  PLL2/2 -> Terminator2/1
  PLL1/2 -> Terminator1/1
  PLL/2 -> Terminator/1
  [Vc] -> PLL2/1
  [Vb] -> PLL1/1
  [Va] -> PLL/1
  Discrete Derivative/1 -> Display1/1, Phasors_dtfreq1/1
  Mux3/1 -> Mux/2
  Mux2/1 -> Mux/1
  Demux1/2 -> [Vb]
  Measurements1/1 -> Demux1/1
  [Va] -> Fourier2/1
  Demux1/3 -> [Vc]
  Demux1/1 -> [Va]
  Mux7/1 -> Mux/5
  Mux4/1 -> Mux/3
  Mux/1 -> Phasors_60Hz/1
  Demux1/4 -> [Ia]
  Demux1/6 -> [Ic]
  Demux1/5 -> [Ib]
  Mux8/1 -> Mux/6
  Mux6/1 -> Mux/4
  Sum of Elements/1 -> Divide/1
  Divide/1 -> Display/1, Discrete Derivative/1, Phasors_freq/1
  Constant/1 -> Divide/2
  Fourier2/2 -> Mux2/2
  [Vc] -> Fourier3/1
  [Ia] -> Fourier4/1
  Fourier2/1 -> Gain/1
  Gain/1 -> Mux2/1
  [Vb] -> Fourier1/1
  Fourier1/2 -> Mux3/2
  Fourier1/1 -> Gain1/1
  Gain1/1 -> Mux3/1
  Fourier3/2 -> Mux4/2
  Fourier3/1 -> Gain2/1
  Gain2/1 -> Mux4/1
  Fourier4/2 -> Mux6/2
  Fourier4/1 -> Gain3/1
  Gain3/1 -> Mux6/1
  Fourier5/2 -> Mux7/2
  Fourier5/1 -> Gain4/1
  Gain4/1 -> Mux7/1
  Fourier6/2 -> Mux8/2
  Fourier6/1 -> Gain5/1
  Gain5/1 -> Mux8/1
  [Ic] -> Fourier6/1
  [Ib] -> Fourier5/1

== system ng_pv_dynamic_dbus_p_4_ss_pmu/SS_PMU/Subsystem8/Subsystem/Subsystem1/Degree to radian1 ==
  Degree : Inport
  Constant : Constant  Value=pi
  Constant1 : Constant  Value=180
  Divide : Product  Inputs=*/
  Product : Product  RndMeth=Zero
  Radian : Outport
  wires:
  Divide/1 -> Radian/1
  Degree/1 -> Product/1
  Constant1/1 -> Divide/2
  Product/1 -> Divide/1
  Constant/1 -> Product/2

== system ng_pv_dynamic_dbus_p_4_ss_pmu/SS_PMU/Subsystem8/Subsystem/Subsystem1/Subsystem ==
  Measurements1 : Inport
  Constant : Constant  Value=3
  Constant{1..5} (5 alike) : Constant  Value=0
  Demux1 : Demux  Outputs=2
  Discrete Derivative : simulink/Discrete/Discrete Derivative  gainval=1.0  ICPrevScaledInput=0.0  InputProcessing=Inherited  OutMin=[]  OutMax=[]  OutDataType=fixdt(1, 16)  OutScaling=2^-10  DoSatur=off
  Display : Display
  Display1 : Display
  Divide : Product  Inputs=*/
  Fourier2 : powerlib_meascontrol/Measurements/Fourier  Freq=60  n=1  InInit=[0, 0]  Ts=Ts
  Fourier4 : powerlib_meascontrol/Measurements/Fourier  Freq=60  n=1  InInit=[0, 0]  Ts=Ts
  Gain : Gain  Gain=1/sqrt(2)
  Gain3 : Gain  Gain=1/sqrt(2)
  Mux : Mux  Inputs=6
  Mux{2..4,6..8} (6 alike) : Mux  Inputs=2
  Mux5 : Mux  Inputs=3
  PLL : powerlib_meascontrol/PLL/PLL  Fmin=60  Par_Init=[0, 60]  ParK=[180, 3200, 1]  TcD=1.6e-4  MaxRateChangeFreq=12  FilterCutOffFreq=25  Ts=Ts  AGC=on
  Sum of Elements : Sum  Inputs=+
  Terminator : Terminator
  Phasors_60Hz : Outport
  Phasors_freq : Outport  Port=2
  Phasors_dtfreq1 : Outport  Port=3
  wires:
  Mux5/1 -> Sum of Elements/1
  PLL/1 -> Mux5/1
  PLL/2 -> Terminator/1
  [Va] -> PLL/1
  Discrete Derivative/1 -> Display1/1, Phasors_dtfreq1/1
  Mux3/1 -> Mux/2
  Mux2/1 -> Mux/1
  Measurements1/1 -> Demux1/1
  [Va] -> Fourier2/1
  Demux1/1 -> [Va]
  Mux7/1 -> Mux/5
  Mux4/1 -> Mux/3
  Mux/1 -> Phasors_60Hz/1
  Demux1/2 -> [Ia]
  Mux8/1 -> Mux/6
  Mux6/1 -> Mux/4
  Sum of Elements/1 -> Divide/1
  Divide/1 -> Display/1, Discrete Derivative/1, Phasors_freq/1
  Constant/1 -> Divide/2
  Fourier2/2 -> Mux2/2
  [Ia] -> Fourier4/1
  Fourier2/1 -> Gain/1
  Gain/1 -> Mux2/1
  Constant4/1 -> Mux3/2, Mux3/1
  Constant5/1 -> Mux4/2, Mux4/1
  Fourier4/2 -> Mux6/2
  Fourier4/1 -> Gain3/1
  Gain3/1 -> Mux6/1
  Constant2/1 -> Mux7/2, Mux7/1
  Constant3/1 -> Mux8/2, Mux8/1
  Constant1/1 -> Mux5/2, Mux5/3

== system ng_pv_dynamic_dbus_p_4_ss_pmu/SS_PMU/Subsystem9/Subsystem/Subsystem1/Degree to radian1 ==
  Degree : Inport
  Constant : Constant  Value=pi
  Constant1 : Constant  Value=180
  Divide : Product  Inputs=*/
  Product : Product  RndMeth=Zero
  Radian : Outport
  wires:
  Divide/1 -> Radian/1
  Degree/1 -> Product/1
  Constant1/1 -> Divide/2
  Product/1 -> Divide/1
  Constant/1 -> Product/2

== system ng_pv_dynamic_dbus_p_4_ss_pmu/SS_PMU/Subsystem9/Subsystem/Subsystem1/Subsystem ==
  Measurements1 : Inport
  Constant : Constant  Value=3
  Demux1 : Demux  Outputs=6
  Discrete Derivative : simulink/Discrete/Discrete Derivative  gainval=1.0  ICPrevScaledInput=0.0  InputProcessing=Inherited  OutMin=[]  OutMax=[]  OutDataType=fixdt(1, 16)  OutScaling=2^-10  DoSatur=off
  Display : Display
  Display1 : Display
  Divide : Product  Inputs=*/
  Fourier{1..6} (6 alike) : powerlib_meascontrol/Measurements/Fourier  Freq=60  n=1  InInit=[0, 0]  Ts=Ts
  Gain{,1..5} (6 alike) : Gain  Gain=1/sqrt(2)
  Mux : Mux  Inputs=6
  Mux{2..4,6..8} (6 alike) : Mux  Inputs=2
  Mux5 : Mux  Inputs=3
  PLL : powerlib_meascontrol/PLL/PLL  Fmin=60  Par_Init=[0, 60]  ParK=[180, 3200, 1]  TcD=1.6e-4  MaxRateChangeFreq=12  FilterCutOffFreq=25  Ts=Ts  AGC=on
  PLL1 : powerlib_meascontrol/PLL/PLL  Fmin=60  Par_Init=[0, 60]  ParK=[180, 3200, 1]  TcD=1.6e-4  MaxRateChangeFreq=12  FilterCutOffFreq=25  Ts=Ts  AGC=on
  PLL2 : powerlib_meascontrol/PLL/PLL  Fmin=60  Par_Init=[0, 60]  ParK=[180, 3200, 1]  TcD=1.6e-4  MaxRateChangeFreq=12  FilterCutOffFreq=25  Ts=Ts  AGC=on
  Sum of Elements : Sum  Inputs=+
  Terminator : Terminator
  Terminator1 : Terminator
  Terminator2 : Terminator
  Phasors_60Hz : Outport
  Phasors_freq : Outport  Port=2
  Phasors_dtfreq1 : Outport  Port=3
  wires:
  Mux5/1 -> Sum of Elements/1
  PLL2/1 -> Mux5/3
  PLL1/1 -> Mux5/2
  PLL/1 -> Mux5/1
  PLL2/2 -> Terminator2/1
  PLL1/2 -> Terminator1/1
  PLL/2 -> Terminator/1
  [Vc] -> PLL2/1
  [Vb] -> PLL1/1
  [Va] -> PLL/1
  Discrete Derivative/1 -> Display1/1, Phasors_dtfreq1/1
  Mux3/1 -> Mux/2
  Mux2/1 -> Mux/1
  Demux1/2 -> [Vb]
  Measurements1/1 -> Demux1/1
  [Va] -> Fourier2/1
  Demux1/3 -> [Vc]
  Demux1/1 -> [Va]
  Mux7/1 -> Mux/5
  Mux4/1 -> Mux/3
  Mux/1 -> Phasors_60Hz/1
  Demux1/4 -> [Ia]
  Demux1/6 -> [Ic]
  Demux1/5 -> [Ib]
  Mux8/1 -> Mux/6
  Mux6/1 -> Mux/4
  Sum of Elements/1 -> Divide/1
  Divide/1 -> Display/1, Discrete Derivative/1, Phasors_freq/1
  Constant/1 -> Divide/2
  Fourier2/2 -> Mux2/2
  [Vc] -> Fourier3/1
  [Ia] -> Fourier4/1
  Fourier2/1 -> Gain/1
  Gain/1 -> Mux2/1
  [Vb] -> Fourier1/1
  Fourier1/2 -> Mux3/2
  Fourier1/1 -> Gain1/1
  Gain1/1 -> Mux3/1
  Fourier3/2 -> Mux4/2
  Fourier3/1 -> Gain2/1
  Gain2/1 -> Mux4/1
  Fourier4/2 -> Mux6/2
  Fourier4/1 -> Gain3/1
  Gain3/1 -> Mux6/1
  Fourier5/2 -> Mux7/2
  Fourier5/1 -> Gain4/1
  Gain4/1 -> Mux7/1
  Fourier6/2 -> Mux8/2
  Fourier6/1 -> Gain5/1
  Gain5/1 -> Mux8/1
  [Ic] -> Fourier6/1
  [Ib] -> Fourier5/1
